simulink model "model_benchmark_traj_test"  (R2018a)
settings: Solver=FixedStepAuto  StartTime=0.0  StopTime=Tf  FixedStep=Tf/N  RelTol=1e-3
values from neighbouring files (symbols this model uses):
  ae1 = model_identified.Parameters(3).Value    [model_benchmark_init.m]    (also in workspace.mat = 1.36231449822)
  ae2 = model_identified.Parameters(4).Value    [model_benchmark_init.m]    (also in workspace.mat = -0.378717172069)
  at = model_identified.Parameters(7).Value    [model_benchmark_init.m]    (also in workspace.mat = -0.463804529993)
  be = model_identified.Parameters(6).Value    [model_benchmark_init.m]    (also in workspace.mat = 0.116311837295)
  bl = model_identified.Parameters(2).Value    [model_benchmark_init.m]    (also in workspace.mat = 0.103160863637)
  bt = model_identified.Parameters(9).Value    [model_benchmark_init.m]    (also in workspace.mat = 0.962119048974)
  ce = model_identified.Parameters(5).Value    [model_benchmark_init.m]    (also in workspace.mat = 0.04469700002)
  cl = model_identified.Parameters(1).Value    [model_benchmark_init.m]    (also in workspace.mat = 0.202457747385)
  ct = model_identified.Parameters(8).Value    [model_benchmark_init.m]    (also in workspace.mat = 0.00762763482449)
  x0 = [0; 0; 0.1745; 0; -0.1047; 0]    [model_benchmark_init.m]    (also in model_benchmark_ode45.m = [0; 0; 0; 0; 0.1; 0]; workspace.mat = [0 0 0.1745 0 -0.1047 0])
settings Model: Creator=obrusvit  LastModifiedBy=obrusvit

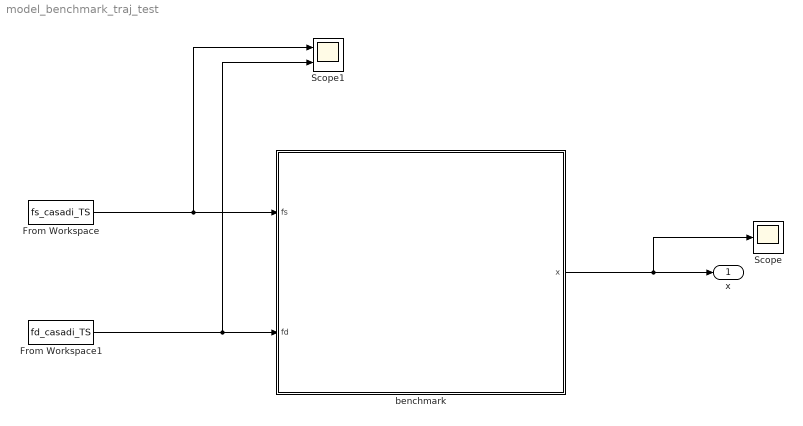
== system model_benchmark_traj_test ==
  From Workspace : FromWorkspace  VariableName=fs_casadi_TS  SampleTime=0
  From Workspace1 : FromWorkspace  VariableName=fd_casadi_TS  SampleTime=0
  Scope : Scope
  Scope1 : Scope  NumInputPorts=2
  benchmark : Subsystem
  x : Outport
  wires:
  benchmark/1(x) -> Scope/1, x/1
  From Workspace1/1 -> Scope1/2, benchmark/2("fd ")
  From Workspace/1 -> Scope1/1, benchmark/1("fs ")

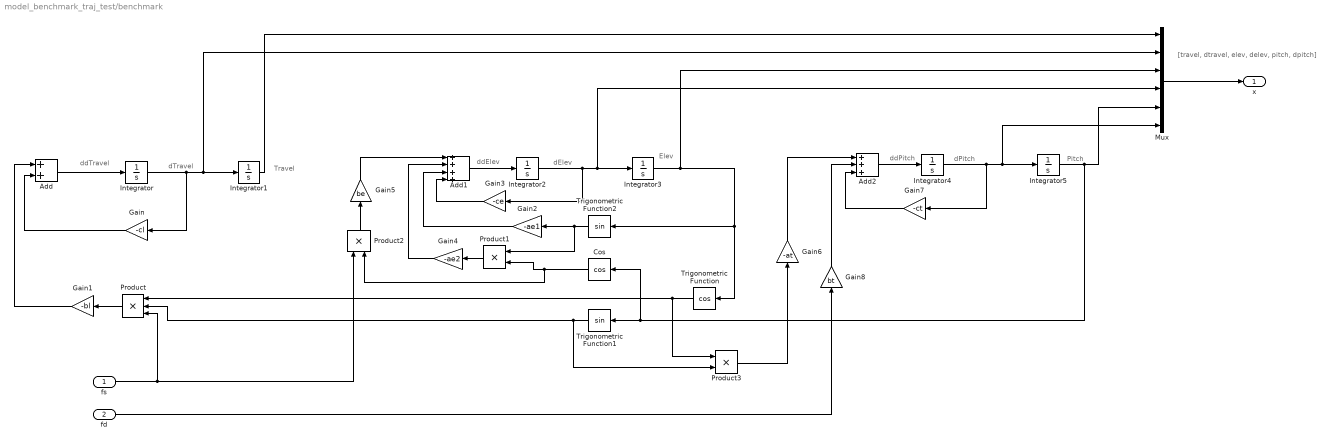
== system model_benchmark_traj_test/benchmark ==
  note: [travel, dtravel, elev, delev, pitch, dpitch]
  note: Pitch
  note: dPitch
  note: ddPitch
  note: Elev
  note: dElev
  note: ddElev
  note: Travel
  note: dTravel
  note: ddTravel
  "fs " : Inport
  "fd " : Inport  Port=2
  Add : Sum
  Add1 : Sum  Inputs=++++
  Add2 : Sum  Inputs=+++
  Cos : Trigonometry  Operator=cos
  Gain : Gain  Gain=-cl
  Gain1 : Gain  Gain=-bl
  Gain2 : Gain  Gain=-ae1
  Gain3 : Gain  Gain=-ce
  Gain4 : Gain  Gain=-ae2
  Gain5 : Gain  Gain=be
  Gain6 : Gain  Gain=-at
  Gain7 : Gain  Gain=-ct
  Gain8 : Gain  Gain=bt
  Integrator : Integrator  InitialCondition=x0(2)
  Integrator1 : Integrator  InitialCondition=x0(1)
  Integrator2 : Integrator  InitialCondition=x0(4)
  Integrator3 : Integrator  InitialCondition=x0(3)
  Integrator4 : Integrator  InitialCondition=x0(6)
  Integrator5 : Integrator  InitialCondition=x0(5)
  Mux : Mux  Inputs=6
  Product : Product  Inputs=3
  Product1 : Product
  Product2 : Product
  Product3 : Product
  Trigonometric Function : Trigonometry  Operator=cos
  Trigonometric Function1 : Trigonometry
  Trigonometric Function2 : Trigonometry
  x : Outport
  wires:
  Gain5/1 -> Add1/1
  Product/1 -> Gain1/1
  Product2/1 -> Gain5/1
  "fd "/1 -> Gain8/1
  Trigonometric Function/1 -> Product3/1, Product/1
  Product3/1 -> Gain6/1
  Gain7/1 -> Add2/3
  Cos/1 -> Product2/2, Product1/2
  Gain4/1 -> Add1/2
  Gain2/1 -> Add1/3
  Mux/1 -> x/1
  Gain8/1 -> Add2/2
  Add2/1 -> Integrator4/1
  Gain6/1 -> Add2/1
  Integrator1/1 -> Mux/1
  Gain1/1 -> Add/1
  Integrator3/1 -> Mux/3, Trigonometric Function2/1, Trigonometric Function/1
  Integrator2/1 -> Gain3/1, Mux/4, Integrator3/1
  Product1/1 -> Gain4/1
  Gain3/1 -> Add1/4
  Integrator4/1 -> Gain7/1, Mux/6, Integrator5/1
  Integrator/1 -> Gain/1, Integrator1/1, Mux/2
  Gain/1 -> Add/2
  Add1/1 -> Integrator2/1
  Integrator5/1 -> Cos/1, Trigonometric Function1/1, Mux/5
  Trigonometric Function2/1 -> Product1/1, Gain2/1
  Trigonometric Function1/1 -> Product3/2, Product/2
  "fs "/1 -> Product2/1, Product/3
  Add/1 -> Integrator/1
